simulink library "DQN_Lib (conflicted copy 2023-11-25 154811)"  (R2023b)
settings: Solver=VariableStepAuto  StartTime=0.0  StopTime=10.0  RelTol=1e-3
undefined symbols (not defined in the file): FreqRad, HrmOrd, Init, La, N, R, Ra, TimeStep, Ts, Ts_dqn, Ws
libraries: $bdroot x4, spsMeanVariableFrequencyLib x4, eeTransforms x3, spsabctodq0Lib x2, spsAlphaBetaZerotodq0Lib x1
(part 1 of 8)
settings Model: Creator=Robert  LastModifiedBy=rober
settings DebuggingCC: UnconnectedInputMsg=warning  UnconnectedOutputMsg=warning  UnconnectedLineMsg=warning
settings ModelReferenceCC: EnableRefExpFcnMdlSchedulingChecks=on
settings RTWCC: DLArmComputeVersion=19.05

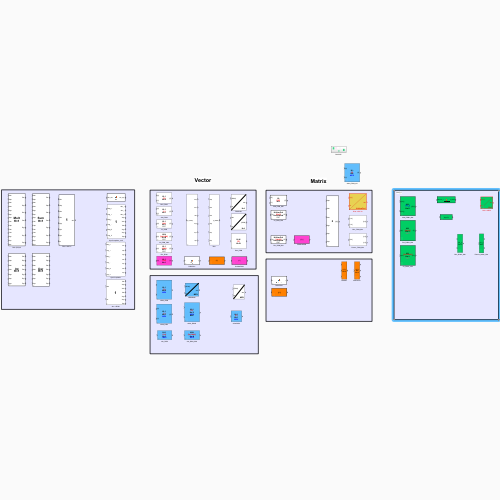
[thumbnail: Simulink's stored preview of the top-level diagram]
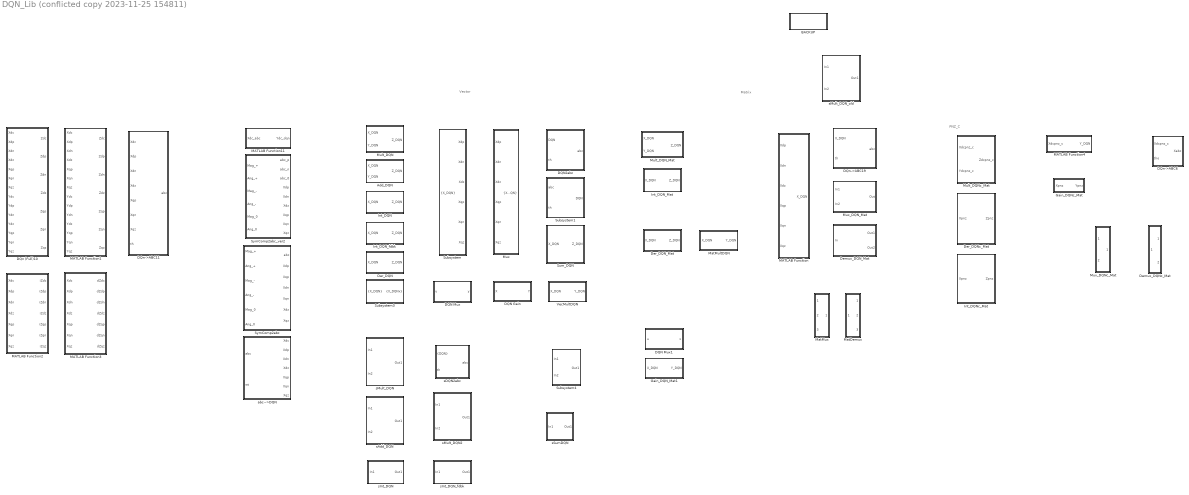
== system DQN_Lib (conflicted copy 2023-11-25 154811) ==
  note: PNZ_C
  note: Vector
  note: Matrix
  Add_DQN : Subsystem  mask{HrmOrd=1, chkHrmLst=off, HrmLst=[1]}
      mask prompts: HrmOrd "Harmonic order:"; chkHrmLst "Only specific harmonics"; HrmLst "Harmonic list:"
      mask Callback chkHrmLst:
      | EMT = get_param(gcb,'chkHrmLst');
      | 
      | if(strcmp(EMT,'on'))
      |    set_param(gcb,'MaskVisibilities',{'on','on','on'});
      | else
      |    set_param(gcb,'MaskVisibilities',{'on','on','off'});
      | end
      mask Display:
      | %plot([0 1])
      | port_label('input',1,'{X}');
      | port_label('input',2,'{Y}');
      | port_label('output',1,'{Z}');
      | 
      | 
      | 
      | harm = get_param(gcb, 'HrmOrd');
      | disp(['{\color{black}\bf\fontsize{12}Hi:',(harm),'}',newline,'{\color{red}\bf\fontsize{12}\{+\}}',newline,'{\color{black}\bf\fontsize{12}Ho:',(harm),'}'], 'texmode','on');
  BACKUP : Subsystem
  DQN Gain : MATLAB Function  TreatAsAtomicUnit=on  mask{H=1, Rvec=[]}
      mask prompts: H "Harmonic order:"; Rvec "[Ca,Cb,Cc]"
  DQN Mux : MATLAB Function  TreatAsAtomicUnit=on  mask{N=1}
      mask prompts: N "Harmonic order:"
  DQN Mux1 : MATLAB Function  TreatAsAtomicUnit=on  mask{N=1}
      mask prompts: N "Harmonic order:"
  DQN2abc : Subsystem  mask{HrmOrd=1}
      mask prompts: HrmOrd "Harmonic order:"
      mask Display:
      | plot([0 1], [0,1])
      | port_label('input',1,'{DQN}');
      | port_label('input',2,'wt');
      | port_label('output',1,'abc');
      | 
      | 
      | 
      | harm = get_param(gcb, 'HrmOrd');
      | %disp([newline,'{\bf\fontsize{12}H=',harm,'}'], 'texmode','on');
      | text(.95,.05,[newline,'{\bf\fontsize{12}H=',harm,'}'], 'horizontalAlignment', 'right', 'verticalAlignment','bottom','texmode','on')
  DQn (Full)10 : MATLAB Function  TreatAsAtomicUnit=on  mask{N=1}
      mask prompts: N "Harmonic order:"
  DQn->ABC11 : MATLAB Function  TreatAsAtomicUnit=on  mask{N=1}
      mask prompts: N "Harmonic order:"
  DQn->ABC19 : MATLAB Function  TreatAsAtomicUnit=on  mask{N=HrmOrd}
      mask prompts: N "Harmonic order:"
  DQn->ABC6 : MATLAB Function  TreatAsAtomicUnit=on  mask{N=1}
      mask prompts: N "Harmonic order:"
  Demux_DQN_Mat : Subsystem  mask{nrOut=2, N=0}
      mask prompts: nrOut "Number of outputs:"; N "Harmonic order:"
      mask init:
      | %fieldnames(get_param('DQn_ABC_Test_compact/Mux34','DialogParameters'))
      | 
      | if(nrOut==0)
      |     Simulink.SubSystem.deleteContents(gcb);
      | else
      | 
      |     PortHandles = get_param(gcb,'PortHandles');
      |     lenInp = length(PortHandles.Outport);
      |     
      |     if(nrOut ~= lenInp)
      | 
      | %         ss_size = ['[6,',num2str(nrOut),'*(',num2str(N+1),')]' ];
      | %         in_size = ['[',num2str(N+1),',6]'];
      | %         out_size = ['[',num2str(nrOut*(N+1)),',6]'];
      |         
      |         out_size = ['[',num2str(N+1),',6]' ];
      |         in_size = ['[',num2str(nrOut*(N+1)),',6]'];
      |         ss_size = ['[6,',num2str(N+1),']' ];
      |         
      |               
      |         Simulink.SubSystem.deleteContents(gcb);
      |         
      |         InportName = 'In';
      |         add_block('built-in/Inport',[gcb,'/',InportName] );
      |         set_param([gcb,'/', InportName ],'position' , [50,65+1*50,90,85+1*50]);
      |                
      |         add_block('simulink/Signal Attributes/Signal Specification', [gcb,'/','Sp_out'], 'Dimensions', in_size );
      |         set_param([gcb,'/','Sp_out'],'position' , [50,65+1*50,90,85+1*50]+[100,0,100,0]);
      |         
      |         add_block('simulink/Quick Insert/Math Operations/Transpose', [gcb,'/Transpose']);
      |         set_param([gcb,'/Transpose'],'position' , [50,65+1*50,90,85+1*50]+[200,0,200,0]);
      |         
      |         add_block('simulink/Math Operations/Reshape', [gcb,'/ss_block'])
      |         set_param([gcb,'/ss_block'],'position' , [50,65+1*50,90,85+1*50]+[300,0,300,0]);
      |        
      |         add_block('built-in/Demux',[gcb,'/Demux'], 'Outputs',num2str(nrOut));
      |         set_param([gcb,'/Demux'],'position' , [200,100,210,100+nrOut*50]+1*[300,0,300,0])
      |         
      |         add_line(gcb,'In/1', 'Sp_out/1','autorouting','on');
      |         add_line(gcb,'Sp_out/1', 'Transpose/1','autorouting','on');
      |         add_line(gcb,'Transpose/1', 'ss_block/1','autorouting','on');
      |         add_line(gcb,'ss_block/1', 'Demux/1','autorouting','on');
      |         
      |         MuxInputs = ['['];
      | 
      |         for i = 1 : nrOut
      |             MuxInputs = [MuxInputs,num2str((N+1)*6),','];
      |             OutportName = strcat('Out',num2str(i));
      |             ReshapeName = strcat('Re_out',num2str(i));
      |             TransposeName = strcat('Tr_out',num2str(i));
      |             SignalSpecName = strcat('Sp_out',num2str(i));
      | 
      |             add_block('built-in/Outport',[gcb,'/',OutportName] );
      |             set_param([gcb,'/', OutportName ],'position' , [750,65+i*50,790,85+i*50]+4*[100,0,100,0]);
      |                        
      |             add_block('simulink/Math Operations/Reshape',[gcb,'/',ReshapeName ], 'OutputDimensionality', 'Customize', 'OutputDimensions',ss_size );
      |             set_param([gcb,'/',ReshapeName ],'position' , [750,65+i*50,790,85+i*50]+1*[100,0,100,0]);
      |             
      |             add_block('simulink/Quick Insert/Math Operations/Transpose', [gcb,'/',TransposeName] );
      |             set_param([gcb,'/',TransposeName],'position' , [750,65+i*50,790,85+i*50]+2*[100,0,100,0]);
      |             
      |             add_block('simulink/Signal Attributes/Signal Specification', [gcb,'/',SignalSpecName], 'Dimensions', out_size );
      |             set_param([gcb,'/',SignalSpecName],'position', [750,65+i*50,790,85+i*50]+3*[100,0,100,0]);
      | 
      |             add_line(gcb,strcat('Demux/',num2str(i)), strcat(ReshapeName,'/1'), 'autorouting','on');
      |             add_line(gcb,strcat(ReshapeName,'/1'), strcat(TransposeName,'/1'),'autorouting','on');
      |             add_line(gcb,strcat(TransposeName,'/1'),strcat(SignalSpecName,'/1'),'autorouting','on');
      |             add_line(gcb,strcat(SignalSpecName,'/1'),strcat(OutportName,'/1'),'autorouting','on');
      |         end
      | 
      |         MuxInputs = [MuxInputs(1:end-1),']'];
      |         set_param([gcb,'/Demux'],'Outputs', MuxInputs);
      |         
      | 
      | 
      |     end
      | end
      mask Display:
      | NN = get_param(gcb, 'N');
      | 
      | 
      | Test = str2num(get_param(gcb, 'N'));
      | 
      | if(isempty(Test))
      |     std = ['[(N+1),6]'];
      |     text = [];
      |     for i = 1 : nrOut
      |         port_label('output',i,std);
      |     end
      |     port_label('input',1,['[',num2str(nrOut),'*(N+1),6]']);
      | else
      |     harm = str2num(NN);
      |     std = ['[',num2str(harm+1),',6]'];
      |     text = [];
      |     for i = 1 : nrOut
      |         port_label('output',i,std);
      |     end
      |     port_label('input',1,['[',num2str(nrOut*(harm+1)),',6]']);
      | end
  Demux_DQNc_Mat : Subsystem  mask{nrOut=2}
      mask prompts: nrOut "Number of outputs [{C}]"
      mask init:
      | if(isempty(nrOut))
      |     Simulink.SubSystem.deleteContents(gcb);
      | else
      | 
      |     IndexOptionArray = cell(2,1);
      |     IndexOptionArray(1) = {'Select all'           };
      |     IndexOptionArray(2) = {'Index vector (dialog)'};
      | 
      |     PortHandles = get_param(gcb,'PortHandles');
      | 
      |     lenOut = length(PortHandles.Outport);
      | 
      |     if(nrOut ~= lenOut) % Important to avoid reinitialization of the block!
      | 
      |         Simulink.SubSystem.deleteContents(gcb);
      | 
      |         add_block('built-in/Inport',[gcb,strcat('/In',num2str(1))]);
      |         set_param([gcb,strcat('/In',num2str(1))],'position' , [50,65+1*50,90,85+1*50]);
      | 
      |         for i = 1 : nrOut
      |             add_block('simulink/Signal Routing/Selector',[gcb,strcat('/Sel',num2str(i))],...
      |                 'IndexOptionArray',IndexOptionArray,...
      |                 'NumberOfDimensions','2',...
      |                 'IndexOptions','Index vector (dialog),Select all',...
      |                 'Indices',strcat(num2str((i-1)*3+1),':',num2str((i-1)*3+3),', 1') ...
      |                 );
      |             set_param([gcb,strcat('/Sel',num2str(i))],'position' , [450,65+i*50,490,85+i*50])
      | 
      | 
      |             add_block('built-in/Outport',[gcb,strcat('/Out',num2str(i))]);
      |             set_param([gcb,strcat('/Out',num2str(i))],'position' , [750,65+i*50,790,85+i*50]);
      | 
      |             add_line(gcb,strcat('In',num2str(1),'/1'),  strcat('Sel',num2str(i),'/1'),'autorouting','on');
      |             add_line(gcb,strcat('Sel',num2str(i),'/1'), strcat('Out',num2str(i),'/1'),'autorouting','on');
      |         end
      | 
      |     end
      | 
      | end
      mask Display: disp(['{\color{red}\bf\fontsize{12}} [\{X_C\}]',newline,' MUX'], 'texmode','on');
  Der_DQN : Subsystem  mask{HrmOrd=1, FreqRad=2*pi*50, Ts=0, EMT=on, sw_soft=on, chkHrmLst=off, HrmLst=[1]}
      mask prompts: HrmOrd "Harmonic order:"; FreqRad "Angular frequency (rad/s);"; Ts "Time step (s):"; EMT "Enable EMT"; sw_soft "Soft start"; chkHrmLst "Only specific harmonics"; HrmLst "Harmonic list:"
      mask Callback EMT:
      | EMT = get_param(gcb,'EMT');
      | EMT2 = get_param(gcb,'chkHrmLst');
      | 
      | 
      | if(strcmp(EMT,'on') && strcmp(EMT2,'on'))
      |    set_param(gcb,'MaskVisibilities',{'on','on','on','on','on','on','on'});
      | elseif(strcmp(EMT,'on') && strcmp(EMT2,'off'))
      |    set_param(gcb,'MaskVisibilities',{'on','on','on','on','on','on','off'});
      | elseif(strcmp(EMT,'off') && strcmp(EMT2,'on'))
      |    set_param(gcb,'MaskVisibilities',{'on','on','on','on','off','on','on'});
      | else
      |    set_param(gcb,'MaskVisibilities',{'on','on','on','on','off','on','off'});
      | end
      mask Callback chkHrmLst:
      | EMT = get_param(gcb,'EMT');
      | EMT2 = get_param(gcb,'chkHrmLst');
      | 
      | 
      | if(strcmp(EMT,'on') && strcmp(EMT2,'on'))
      |    set_param(gcb,'MaskVisibilities',{'on','on','on','on','on','on','on'});
      | elseif(strcmp(EMT,'on') && strcmp(EMT2,'off'))
      |    set_param(gcb,'MaskVisibilities',{'on','on','on','on','on','on','off'});
      | elseif(strcmp(EMT,'off') && strcmp(EMT2,'on'))
      |    set_param(gcb,'MaskVisibilities',{'on','on','on','on','off','on','on'});
      | else
      |    set_param(gcb,'MaskVisibilities',{'on','on','on','on','off','on','off'});
      | end
      mask Display:
      | %plot([0 1])
      | port_label('input',1,'{X}');
      | port_label('output',1,'{Z}');
      | 
      | harm = get_param(gcb, 'HrmOrd');
      | 
      | if(numel(get_param(gcb, 'EMT'))==2)
      |     disp(['{\color{black}\bf\fontsize{12}Hi:',(harm),'}',newline,'{\color{red}\bf\fontsize{12}\{d/dt\}}',newline,'{\color{black}\bf\fontsize{12}Ho:',(harm),'}',newline,'{\color{gray}\bf\fontsize{12}EMT}'], 'texmode','on');
      | else
      |     disp(['{\color{black}\bf\fontsize{12}Hi:',(harm),'}',newline,'{\color{red}\bf\fontsize{12}\{d/dt\}}',newline,'{\color{black}\bf\fontsize{12}Ho:',(harm),'}'], 'texmode','on');
      | end
  Der_DQN_Mat : MATLAB Function  TreatAsAtomicUnit=on  mask{N=HrmOrd, w=FreqRad, Ts=Ts, EMT=on, sw_soft=on}
      mask prompts: N "Harmonic order:"; w "Frequency (rad/s):"; Ts "Time step (s):"; EMT "Enable EMT"; sw_soft "Soft start?"
  Der_DQNc_Mat : MATLAB Function  TreatAsAtomicUnit=on  mask{Ts=50e-6, N=1, w=2*pi*50, EMT=on, sw_soft=on}
      mask prompts: Ts "Time step (s):"; N "Harmonic order:"; w "Angular frequency [1/rad]:"; sw_soft "Soft start"
  Gain_DQN_Mat1 : MATLAB Function  TreatAsAtomicUnit=on  mask{H=1, R=[], chkInv=off}
      mask prompts: H "Harmonic order:"; R "Line matrix [3x3]"; chkInv "Invert?"
  Gain_DQNc_Mat : MATLAB Function  TreatAsAtomicUnit=on  mask{Rabc=[R zeros(3,3); zeros(3,3) R], HRM=N, chkInv=off}
      mask prompts: Rabc "Line matrix [3x3]:"; HRM "Harmonic order:"; chkInv "Invert"
  Int_DQN : Subsystem  mask{HrmOrd=1, FreqRad=2*pi*50, TimeStep=50e-6, Init=zeros(1,6), EMT=on, chkHrmLst=off, HrmLst=[1]}
      mask prompts: HrmOrd "Harmonic order:"; FreqRad "Angular frequency (rad/s);"; TimeStep "Time step (s):"; Init "DC init [1x6]:"; EMT "Enable EMT"; chkHrmLst "Only specific harmonics"; HrmLst "Harmonic list:"
      mask Callback chkHrmLst:
      | EMT = get_param(gcb,'chkHrmLst');
      | 
      | if(strcmp(EMT,'on'))
      |    set_param(gcb,'MaskVisibilities',{'on','on','on','on','on','on','on'});
      | else
      |    set_param(gcb,'MaskVisibilities',{'on','on','on','on','on','on','off'});
      | end
      mask Display:
      | %plot([0 1])
      | port_label('input',1,'{X}');
      | port_label('output',1,'{Z}');
      | 
      | harm = get_param(gcb, 'HrmOrd');
      | 
      | if(numel(get_param(gcb, 'EMT'))==2)
      |     disp(['{\color{black}\bf\fontsize{12}Hi:',(harm),'}',newline,'{\color{red}\bf\fontsize{12}\{Int\}}',newline,'{\color{black}\bf\fontsize{12}Ho:',(harm),'}',newline,'{\color{gray}\bf\fontsize{12}EMT}'], 'texmode','on');
      | else
      |     disp(['{\color{black}\bf\fontsize{12}Hi:',(harm),'}',newline,'{\color{red}\bf\fontsize{12}\{Int\}}',newline,'{\color{black}\bf\fontsize{12}Ho:',(harm),'}'], 'texmode','on');
      | end
  Int_DQN_Mat : MATLAB Function  TreatAsAtomicUnit=on  mask{N=HrmOrd, dt=TimeStep, w=FreqRad, EMT=on, InitInt=Init}
      mask prompts: N "Order number:"; dt "Time step (s):"; w "Angular frequency (1/rad):"; InitInt "Initial conditions [1x6]:"
  Int_DQN_fdbk : Subsystem  mask{HrmOrd=N, FreqRad=Ws, TimeStep=Ts_dqn, swFeed=on, R=Ra, iL=1/La}
      mask prompts: HrmOrd "Harmonic order:"; FreqRad "Angular frequency (rad/s);"; TimeStep "Time step (s):"; swFeed "Enable feedback"; R "Feedback parameter (Kr):"; iL "Integrator parameter (Kl):"
      mask Callback swFeed:
      | EMT = get_param(gcb,'swFeed');
      | 
      | if(strcmp(EMT,'on'))
      |    set_param(gcb,'MaskVisibilities',{'on','on','on','on','on','on'});
      | else
      |    set_param(gcb,'MaskVisibilities',{'on','on','on','on','off','off'});
      | end
      mask Display:
      | %plot([0 1])
      | port_label('input',1,'{X}');
      | port_label('output',1,'{Z}');
      | 
      | harm = get_param(gcb, 'HrmOrd');
      | disp(['{\color{black}\bf\fontsize{12}Hi:',(harm),'}',newline,'{\color{red}\bf\fontsize{12}\{Int-fdbk\}}',newline,'{\color{black}\bf\fontsize{12}Ho:',(harm),'}',newline,'{\color{gray}\bf\fontsize{12}EMT}'], 'texmode','on');
  Int_DQNc_Mat : MATLAB Function  TreatAsAtomicUnit=on  mask{N=1, dt=50e-6, w=2*pi*50, InitInt=zeros(3,1), swFeed=on, R=eye(3), iL=eye(3)}
      mask prompts: N "Order number:"; dt "Time step (s):"; w "Angular frequency (1/rad):"; InitInt "Initial conditions DC [3x1]:"; swFeed "Enable feedback"; R "Feedback parameter (Kr {abc}):"; iL "Feedback parameter (Ki {abc}):"
  MATLAB Function : MATLAB Function  TreatAsAtomicUnit=on  mask{N=0}
      mask prompts: N "Harmonic order:"
  MATLAB Function1 : MATLAB Function  TreatAsAtomicUnit=on  mask{N=1}
      mask prompts: N "Harmonic order:"
  MATLAB Function11 : MATLAB Function  TreatAsAtomicUnit=on
  MATLAB Function2 : MATLAB Function  TreatAsAtomicUnit=on  mask{N=1, w=2*pi*50, Ts=50e-6, IntDC=on}
      mask prompts: N "Harmonic order:"; w "Frequency (rad/s):"; Ts "Time step (s):"; IntDC "Integrate Xdc?"
  MATLAB Function3 : MATLAB Function  TreatAsAtomicUnit=on  mask{N=1, w=2*pi*50, Ts=0, EMT=0}
      mask prompts: N "Harmonic order:"; w "Frequency (rad/s):"; Ts "Time step (s):"; EMT "Enable EMT"
  MATLAB Function4 : MATLAB Function  TreatAsAtomicUnit=on
  MatDemux : Subsystem  mask{nrOut=3}
      mask prompts: nrOut "Number of outputs [{C}]"
      mask init:
      | if(isempty(nrOut))
      |     Simulink.SubSystem.deleteContents(gcb);
      | else
      | 
      |     IndexOptionArray = cell(2,1);
      |     IndexOptionArray(1) = {'Select all'           };
      |     IndexOptionArray(2) = {'Index vector (dialog)'};
      | 
      |     PortHandles = get_param(gcb,'PortHandles');
      | 
      |     lenOut = length(PortHandles.Outport);
      | 
      |     if(nrOut ~= lenOut) % Important to avoid reinitialization of the block!
      | 
      |         Simulink.SubSystem.deleteContents(gcb);
      | 
      |         add_block('built-in/Inport',[gcb,strcat('/In',num2str(1))]);
      |         set_param([gcb,strcat('/In',num2str(1))],'position' , [50,65+1*50,90,85+1*50]);
      | 
      |         for i = 1 : nrOut
      |             add_block('simulink/Signal Routing/Selector',[gcb,strcat('/Sel',num2str(i))],...
      |                 'IndexOptionArray',IndexOptionArray,...
      |                 'NumberOfDimensions','2',...
      |                 'IndexOptions','Select all,Index vector (dialog)',...
      |                 'Indices',strcat('1,',num2str((i-1)*6+1),':',num2str((i-1)*6+6)) );
      |             set_param([gcb,strcat('/Sel',num2str(i))],'position' , [450,65+i*50,490,85+i*50])
      | 
      | 
      |             add_block('built-in/Outport',[gcb,strcat('/Out',num2str(i))]);
      |             set_param([gcb,strcat('/Out',num2str(i))],'position' , [750,65+i*50,790,85+i*50]);
      | 
      |             add_line(gcb,strcat('In',num2str(1),'/1'),  strcat('Sel',num2str(i),'/1'),'autorouting','on');
      |             add_line(gcb,strcat('Sel',num2str(i),'/1'), strcat('Out',num2str(i),'/1'),'autorouting','on');
      |         end
      | 
      |     end
      | 
      | end
      mask Display: disp(['{\color{red}\bf\fontsize{12}} [\{C\}]',newline,'  DE-',newline,' MUX'], 'texmode','on');
  MatMultDQN : MATLAB Function  TreatAsAtomicUnit=on  mask{H=1, R=[], chkInv=off}
      mask prompts: H "Harmonic order:"; R "Line matrix [3x3]"; chkInv "Invert?"
  MatMux : Subsystem  mask{nrInp=3}
      mask prompts: nrInp "Number of inputs [{C}]"
      mask init:
      | %blocks = find_system(gcb,'LookUnderMasks','on','FollowLinks','on')
      | %set_param(gcb, 'MaskSelfModifiable', 'on');
      | 
      | % if(SSM == [])
      | %     Simulink.SubSystem.deleteContents(gcb);
      | % else
      | 
      | if(isempty(nrInp))
      |     Simulink.SubSystem.deleteContents(gcb);
      | else
      | 
      |     nrOut = 1;
      | 
      | 
      | PortHandles = get_param(gcb,'PortHandles');
      | lenInp = length(PortHandles.Inport);
      | lenOut = length(PortHandles.Inport);
      | 
      | if(nrInp ~= lenInp)
      |     %disp('ENTERED')
      |     Simulink.SubSystem.deleteContents(gcb);
      | %     add_block('simulink/Continuous/State-Space', [gcb,'/ss_block'], 'A','SS.A', 'B','SS.B', 'C','SS.C', 'D','SS.D', 'X0','X0')
      | %     set_param([gcb,'/ss_block'],'position' , [350,100,450,150])
      | 
      | 
      | 
      |         add_block('simulink/Math Operations/Matrix Concatenate',[gcb,'/Mux'], 'NumInputs',num2str(nrInp), 'ConcatenateDimension',num2str(2));
      |         set_param([gcb,'/Mux'],'position' , [200,100,250,100+nrInp*50])
      |         
      | %         add_block('built-in/Demux',[gcb,'/Demux'], 'Outputs',num2str(nrOut));
      | %         set_param([gcb,'/Demux'],'position' , [500,100,550,100+nrOut*50])
      | 
      | 
      |         for i = 1 : nrInp
      |             add_block('built-in/Inport',[gcb,strcat('/In',num2str(i))]);
      |             set_param([gcb,strcat('/In',num2str(i))],'position' , [50,65+i*50,90,85+i*50]);
      |             add_line(gcb,strcat('In',num2str(i),'/1'),strcat('Mux/',num2str(i)),'autorouting','on');
      |         end
      | 
      |         for i = 1 : nrOut
      |             add_block('built-in/Outport',[gcb,strcat('/Out',num2str(i))]);
      |             set_param([gcb,strcat('/Out',num2str(i))],'position' , [750,65+i*50,790,85+i*50]);
      |             add_line(gcb,strcat('Mux/',num2str(i)), strcat('Out',num2str(i),'/1'),'autorouting','on');
      |         end
      | 
      | 
      | %     add_line(gcb, 'Mux/1', 'ss_block/1')
      | %     add_line(gcb, 'ss_block/1', 'Demux/1')
      | 
      | end
      | 
      | end
      mask Display: disp(['{\color{red}\bf\fontsize{12}} [\{C\}]',newline,' MUX'], 'texmode','on');
  Mult_DQN : Subsystem  mask{HrmOrd=1, HrmDbl=on, chkHrmLst=off, HrmLstX=[1], HrmLstY=[1]}
      mask prompts: HrmOrd "Harmonic order:"; HrmDbl "Double harmonic"; chkHrmLst "Only specific harmonics"; HrmLstX "Harmonic list X:"; HrmLstY "Harmonic list Y:"
      mask Callback chkHrmLst:
      | EMT = get_param(gcb,'chkHrmLst');
      | 
      | if(strcmp(EMT,'on'))
      |    set_param(gcb,'MaskVisibilities',{'on','on','on','on','on'});
      | else
      |    set_param(gcb,'MaskVisibilities',{'on','on','on','off','off'});
      | end
      mask Display:
      | %plot([0 1])
      | port_label('input',1,'{X}');
      | port_label('input',2,'{Y}');
      | port_label('output',1,'{Z}');
      | 
      | 
      | 
      | harm = str2num(get_param(gcb, 'HrmOrd'));
      | HrmDbl = get_param(gcb, 'HrmDbl');
      | if(HrmDbl=="on")
      |     disp(['{\color{black}\bf\fontsize{12}Hi:',num2str(harm),'}',newline,'{\color{red}\bf\fontsize{12}\{X\}}',newline,'{\color{black}\bf\fontsize{12}Ho:',num2str(2*harm),'}'], 'texmode','on');
      | else
      |     disp(['{\color{black}\bf\fontsize{12}Hi:',num2str(harm),'}',newline,'{\color{red}\bf\fontsize{12}\{X\}}',newline,'{\color{black}\bf\fontsize{12}Ho:',num2str(harm),'}'], 'texmode','on');
      | end
      | 
      | 
      | %text(.95,.05,[newline,'{\bf\fontsize{12}H=',harm,'}'], 'horizontalAlignment', 'right', 'verticalAlignment','bottom','texmode','on')
  Mult_DQN_Mat : MATLAB Function  TreatAsAtomicUnit=on  mask{N=HrmOrd, HrmDbl=on}
      mask prompts: N "Harmonic order:"; HrmDbl "Double Harmonic"
  Mult_DQNc_Mat : MATLAB Function  TreatAsAtomicUnit=on  mask{N=1, HrmDbl=on}
      mask prompts: N "Harmonic order:"; HrmDbl "Double Harmonic"
  Mux : Subsystem  mask{N=1}
      mask prompts: N "Harmonic order:"
  Mux_DQN_Mat : Subsystem  mask{nrInp=2, N=0}
      mask prompts: nrInp "Number of inputs:"; N "Harmonic order:"
      mask init:
      | %fieldnames(get_param('DQn_ABC_Test_compact/Mux34','DialogParameters'))
      | 
      | if(nrInp==0)
      |     Simulink.SubSystem.deleteContents(gcb);
      | else
      | 
      |     PortHandles = get_param(gcb,'PortHandles');
      |     lenInp = length(PortHandles.Inport);
      |     lenOut = length(PortHandles.Inport);
      |     
      |     if(nrInp ~= lenInp)
      | 
      |         ss_size = ['[6,',num2str(nrInp),'*(',num2str(N+1),')]' ];
      |         in_size = ['[',num2str(N+1),',6]'];
      |         out_size = ['[',num2str(nrInp*(N+1)),',6]'];
      |         
      |         Simulink.SubSystem.deleteContents(gcb);
      |         add_block('simulink/Math Operations/Reshape', [gcb,'/ss_block'], 'OutputDimensionality', 'Customize', 'OutputDimensions', ss_size)
      |         set_param([gcb,'/ss_block'],'position' , [350,100,450,150]+[300,0,300,0])
      | 
      | 
      |         add_block('built-in/Mux',[gcb,'/Mux'], 'Inputs',num2str(nrInp));
      |         set_param([gcb,'/Mux'],'position' , [200,100,250,100+nrInp*50]+[300,0,300,0])
      |         
      |         MuxInputs = ['['];
      | 
      |         for i = 1 : nrInp
      |             MuxInputs = [MuxInputs,num2str((N+1)*6),','];
      |             InportName = strcat('In',num2str(i));
      |             ReshapeName = strcat('Re_in',num2str(i));
      |             TransposeName = strcat('Tr_in',num2str(i));
      |             SignalSpecName = strcat('Sp_in',num2str(i));
      | 
      |             add_block('built-in/Inport',[gcb,'/',InportName] );
      |             set_param([gcb,'/', InportName ],'position' , [50,65+i*50,90,85+i*50]);
      |             
      |             add_block('simulink/Signal Attributes/Signal Specification', [gcb,'/',SignalSpecName], 'Dimensions', in_size );
      |             set_param([gcb,'/',SignalSpecName],'position' , [50,65+i*50,90,85+i*50]+[100,0,100,0]);
      |             
      |             add_block('simulink/Quick Insert/Math Operations/Transpose', [gcb,'/',TransposeName] );
      |             set_param([gcb,'/',TransposeName],'position' , [50,65+i*50,90,85+i*50]+[200,0,200,0]);
      |             
      |             add_block('simulink/Math Operations/Reshape',[gcb,'/',ReshapeName ]);
      |             set_param([gcb,'/',ReshapeName ],'position' , [50,65+i*50,90,85+i*50]+[300,0,300,0]);
      | 
      |             add_line(gcb,strcat(InportName,'/1'), strcat(SignalSpecName,'/1'), 'autorouting','on');
      |             add_line(gcb,strcat(SignalSpecName,'/1'), strcat(TransposeName,'/1'), 'autorouting','on');
      |             add_line(gcb,strcat(TransposeName,'/1'), strcat(ReshapeName,'/1'), 'autorouting','on');
      |             add_line(gcb,strcat(ReshapeName,'/1'),strcat('Mux/',num2str(i)),'autorouting','on');
      | 
      |         end
      |         MuxInputs = [MuxInputs(1:end-1),']'];
      |         set_param([gcb,'/Mux'],'Inputs', MuxInputs);
      |         
      |         add_block('simulink/Signal Attributes/Signal Specification', [gcb,'/','Sp_out'], 'Dimensions', out_size );
      |         set_param([gcb,'/','Sp_out'],'position' , [750,65+1*50,790,85+1*50]+[200,0,200,0]);
      | 
      |         add_block('built-in/Outport',[gcb,'/Out']);
      |         set_param([gcb,'/Out'],'position' , [750,65+1*50,790,85+1*50]+[300,0,300,0]);
      |         add_line(gcb,'Mux/1','ss_block/1','autorouting','on');
      | 
      |         add_block('simulink/Quick Insert/Math Operations/Transpose', [gcb,'/Transpose']);
      |         set_param([gcb,'/Transpose'],'position' , [750,65+1*50,790,85+1*50]+[100,0,100,0]);
      |         
      |         
      |         add_line(gcb,'ss_block/1', 'Transpose/1','autorouting','on');
      |         add_line(gcb,'Transpose/1', 'Sp_out/1','autorouting','on');
      |         add_line(gcb,'Sp_out/1', 'Out/1','autorouting','on');
      | 
      |     end
      | end
      mask Display:
      | NN = get_param(gcb, 'N');
      | 
      | 
      | Test = str2num(get_param(gcb, 'N'));
      | 
      | if(isempty(Test))
      |     std = ['[(N+1),6]'];
      |     text = [];
      |     for i = 1 : nrInp
      |         port_label('input',i,std);
      |     end
      |     port_label('output',1,['[',num2str(nrInp),'*(N+1),6]']);
      | else
      |     harm = str2num(NN);
      |     std = ['[',num2str(harm+1),',6]'];
      |     text = [];
      |     for i = 1 : nrInp
      |         port_label('input',i,std);
      |     end
      |     port_label('output',1,['[',num2str(nrInp*(harm+1)),',6]']);
      | end
  Mux_DQNc_Mat : Subsystem  mask{nrInp=2}
      mask prompts: nrInp "Number of inputs [{C}]"
      mask init:
      | %blocks = find_system(gcb,'LookUnderMasks','on','FollowLinks','on')
      | %set_param(gcb, 'MaskSelfModifiable', 'on');
      | 
      | % if(SSM == [])
      | %     Simulink.SubSystem.deleteContents(gcb);
      | % else
      | 
      | if(isempty(nrInp))
      |     Simulink.SubSystem.deleteContents(gcb);
      | else
      | 
      |     nrOut = 1;
      | 
      | 
      | PortHandles = get_param(gcb,'PortHandles');
      | lenInp = length(PortHandles.Inport);
      | lenOut = length(PortHandles.Inport);
      | 
      | if(nrInp ~= lenInp)
      |     %disp('ENTERED')
      |     Simulink.SubSystem.deleteContents(gcb);
      | %     add_block('simulink/Continuous/State-Space', [gcb,'/ss_block'], 'A','SS.A', 'B','SS.B', 'C','SS.C', 'D','SS.D', 'X0','X0')
      | %     set_param([gcb,'/ss_block'],'position' , [350,100,450,150])
      | 
      | 
      | 
      |         add_block('simulink/Math Operations/Matrix Concatenate',[gcb,'/Mux'], 'NumInputs',num2str(nrInp), 'ConcatenateDimension',num2str(1));
      |         set_param([gcb,'/Mux'],'position' , [200,100,250,100+nrInp*50])
      |         
      | %         add_block('built-in/Demux',[gcb,'/Demux'], 'Outputs',num2str(nrOut));
      | %         set_param([gcb,'/Demux'],'position' , [500,100,550,100+nrOut*50])
      | 
      | 
      |         for i = 1 : nrInp
      |             add_block('built-in/Inport',[gcb,strcat('/In',num2str(i))]);
      |             set_param([gcb,strcat('/In',num2str(i))],'position' , [50,65+i*50,90,85+i*50]);
      |             add_line(gcb,strcat('In',num2str(i),'/1'),strcat('Mux/',num2str(i)),'autorouting','on');
      |         end
      | 
      |         for i = 1 : nrOut
      |             add_block('built-in/Outport',[gcb,strcat('/Out',num2str(i))]);
      |             set_param([gcb,strcat('/Out',num2str(i))],'position' , [750,65+i*50,790,85+i*50]);
      |             add_line(gcb,strcat('Mux/',num2str(i)), strcat('Out',num2str(i),'/1'),'autorouting','on');
      |         end
      | 
      | 
      | %     add_line(gcb, 'Mux/1', 'ss_block/1')
      | %     add_line(gcb, 'ss_block/1', 'Demux/1')
      | 
      | end
      | 
      | end
      mask Display: disp(['{\color{red}\bf\fontsize{12}} [\{X_C\}]',newline,' MUX'], 'texmode','on');
  Subsystem : Subsystem  mask{N=1}
      mask prompts: N "Harmonic order:"
  Subsystem1 : Subsystem  mask{HrmOrd=1, Freq=0, Ts=50e-6}
      mask prompts: HrmOrd "Harmonic order:"; Freq "Frequency (Hz):"; Ts "Sample time (s):"
      mask Display:
      | plot([0 1], [0,1])
      | port_label('input',1,'abc');
      | port_label('input',2,'wt');
      | port_label('output',1,'{DQN}');
      | 
      | 
      | 
      | harm = get_param(gcb, 'HrmOrd');
      | %disp([newline,'{\bf\fontsize{12}H=',harm,'}'], 'texmode','on');
      | text(.95,.05,[newline,'{\bf\fontsize{12}H=',harm,'}'], 'horizontalAlignment', 'right', 'verticalAlignment','bottom','texmode','on')
  Subsystem3 : Subsystem  mask{HOI=1, HOO=1}
      mask prompts: HOI "Input harmonic order:"; HOO "Output harmonic order:"
      mask Display:
      | %plot([0 1])
      | port_label('input',1,'{X}');
      | port_label('output',1,'{Y}');
      | 
      | 
      | 
      | HOI = get_param(gcb, 'HOI');
      | HOO = get_param(gcb, 'HOO');
      | disp(['{\color{black}\bf\fontsize{12}Hi:',(HOI),'}',newline,'{\color{red}\bf\fontsize{12}Trim}',newline,'{\color{black}\bf\fontsize{12}Ho:',(HOO),'}'], 'texmode','on');
  Subsystem4 : Subsystem
      mask Display:
      | plot([0 1], [0,1])
      | port_label('input',1,'{DQN}');
      | port_label('input',2,'wt');
      | port_label('output',1,'abc');
      | 
      | text(.95,.05,[newline,'{\bf\fontsize{12}MEX}'], 'horizontalAlignment', 'right', 'verticalAlignment','bottom','texmode','on')
  Sum_DQN : Subsystem  mask{HrmOrd=N}
      mask prompts: HrmOrd "Harmonic order:"
      mask Display:
      | %plot([0 1])
      | %port_label('input',1,'{X}');
      | %port_label('output',1,'{Z}');
      | 
      | port_label('input',1,'');
      | port_label('output',1,'');
      | 
      | harm = get_param(gcb, 'HrmOrd');
      | disp(['{\color{black}\bf\fontsize{12}Hi:',(harm),'}',newline,'{\color{red}\bf\fontsize{12}\{\Sigma\}}',newline,'{\color{black}\bf\fontsize{12}Ho:',(harm),'}'], 'texmode','on');
      | 
      | radius = 1
      | 
      | 
      | rsq = radius * radius;
      | R = round(radius);
      | c = R + 1;
      | t = 2*R + 1;
      | y = zeros(t);
      | 
      | % points on St George's cross
      | y(:, c) = 1;
      | y(c, :) = 1;
      | 
      | for rstart = 1:R
      |     rend = round(sqrt(rsq - rstart * rstart));
      |     if rend < rstart
      |         break
      |     end
      | 
      |     % points on St Andrew's cross
      |     y(c+rstart, c+rstart) = 1;
      |     y(c+rstart, c-rstart) = 1;
      |     y(c-rstart, c+rstart) = 1;
      |     y(c-rstart, c-rstart) = 1;
      | 
      |     % fill in octants
      |     y(c+rstart:c+rend, c+rstart) = 1;
      |     y(c+rstart:c+rend, c-rstart) = 1;
      |     y(c-rend:c-rstart, c+rstart) = 1;
      |     y(c-rend:c-rstart, c-rstart) = 1;
      |     y(c+rstart, c+rstart:c+rend) = 1;
      |     y(c-rstart, c+rstart:c+rend) = 1;
      |     y(c+rstart, c-rend:c-rstart) = 1;
      |     y(c-rstart, c-rend:c-rstart) = 1;
      | end
  SymComp2abc : Subsystem  mask{H=1, f=50}
      mask prompts: H "Harmonic order:"; f "Frequency (1/s):"
  SymComp2abc_ver2 : Subsystem  mask{H=1, f=50}
      mask prompts: H "Harmonic order:"; f "Frequency (1/s):"
      mask Display:
      | port_label('input',1,'Mag_+');
      | port_label('input',2,'Ang_+');
      | port_label('input',3,'Mag_-');
      | port_label('input',4,'Ang_-');
      | port_label('input',5,'Mag_0');
      | port_label('input',6,'Ang_0');
      | 
      | 
      | port_label('output',1,'abc_+');
      | port_label('output',2,'abc_-');
      | port_label('output',3,'abc_0');
      | port_label('output',4,'Xdp');
      | port_label('output',5,'Xdn');
      | port_label('output',6,'Xdz');
      | port_label('output',7,'Xqp');
      | port_label('output',8,'Xqn');
      | port_label('output',9,'Xqz');
      | 
      | 
      | 
      | harm = get_param(gcb, 'H');
      | disp(['{\bf\fontsize{24}',harm,'}'], 'texmode','on');
  VecMultDQN : MATLAB Function  TreatAsAtomicUnit=on  mask{H=1, R=[], chkInv=off}
      mask prompts: H "Harmonic order:"; R "Line matrix [3x3]"; chkInv "Invert?"
  abc-->DQN : Subsystem  mask{H=1, f=50, Ts=Ts}
      mask prompts: H "Harmonic order:"; f "Frequency (Hz):"; Ts "Sample time (s):"
      mask Display:
      | port_label('input',1,'abc');
      | port_label('input',2,'wt');
      | 
      | port_label('output',1,'Xdc');
      | port_label('output',2,'Xdp');
      | port_label('output',3,'Xdn');
      | port_label('output',4,'Xdz');
      | port_label('output',5,'Xqp');
      | port_label('output',6,'Xqn');
      | port_label('output',7,'Xqz');
      | 
      | 
      | 
      | harm = get_param(gcb, 'H');
      | disp(['{\bf\fontsize{24}',harm,'}'], 'texmode','on');
  sAdd_DQN : Subsystem  mask{HRM=1}
      mask prompts: HRM "Harmonic order:"
      mask Display:
      | %plot([0 1])
      | port_label('input',1,'{X}');
      | port_label('input',2,'{Y}');
      | port_label('output',1,'{Z}');
      | 
      | 
      | 
      | %harm = (get_param(gcb, 'HRM'));
      | %disp(['{\color{black}\bf\fontsize{12}Hi:',num2str(harm),'}',newline,'{\color{red}\bf\fontsize{12}\{+\}}',newline,'{\color{black}\bf\fontsize{12}Ho:',num2str(harm),newline,'{\color{blue}\bf\fontsize{12}MEX}','}'], 'texmode','on');
      | harm = get_param(gcb, 'HRM');
      | disp(['{\color{black}\bf\fontsize{12}Hi:',(harm),'}',newline,'{\color{red}\bf\fontsize{12}\{+\}}',newline,'{\color{black}\bf\fontsize{12}Ho:',(harm),newline,'{\color{blue}\bf\fontsize{12}MEX}','}'], 'texmode','on');
  sDQN2abc : Subsystem  mask{HRM=1}
      mask prompts: HRM "Harmonic order:"
      mask Display:
      | plot([0 1], [0,1])
      | port_label('input',1,'{DQN}');
      | port_label('input',2,'wt');
      | port_label('output',1,'abc');
      | 
      | text(.95,.05,[newline,'{\bf\fontsize{12}MEX}'], 'horizontalAlignment', 'right', 'verticalAlignment','bottom','texmode','on')
  sInt_DQN : Subsystem  mask{HRM=1, Ws=2*pi*50, Ts=50e-6, HrmSeq=off}
      mask prompts: HRM "Harmonic order:"; Ws "Angular frequency (1/rad):"; Ts "Time step (s):"; HrmSeq "Pos. odd / neg. even harmonics (1p, 2n, 3p...)"
      mask Display:
      | %plot([0 1])
      | %port_label('input',1,'{X}');
      | %port_label('output',1,'{Z}');
      | 
      | port_label('input',1,'');
      | port_label('output',1,'');
      | 
      | harm = get_param(gcb, 'HRM');
      | 
      | disp(['{\color{black}\bf\fontsize{12}Hi:',(harm),'}',newline,'{\color{red}\bf\fontsize{12}\{Int\}}',newline,'{\color{black}\bf\fontsize{12}Ho:',(harm),'}',newline,'{\color{blue}\bf\fontsize{12}MEX}'], 'texmode','on');
  sInt_DQN_fdbk : Subsystem  mask{HRM=N, Ws=Ws, Ts=Ts, HrmSeq=off, swFeed=off, R=1, iL=1}
      mask prompts: HRM "Harmonic order:"; Ws "Angular frequency (1/rad):"; Ts "Time step (s):"; HrmSeq "Pos. odd / neg. even harmonics (1p, 2n, 3p...)"; swFeed "Enable feedback"; R "Feedback parameter (Kr):"; iL "Integrator parameter (Ki):"
      mask Callback swFeed:
      | EMT = get_param(gcb,'swFeed');
      | 
      | if(strcmp(EMT,'on'))
      |    set_param(gcb,'MaskVisibilities',{'on','on','on','on','on','on','on'});
      | else
      |    set_param(gcb,'MaskVisibilities',{'on','on','on','on','on','off','off'});
      | end
      mask Display:
      | %plot([0 1])
      | %port_label('input',1,'{X}');
      | %port_label('output',1,'{Z}');
      | 
      | port_label('input',1,'');
      | port_label('output',1,'');
      | 
      | harm = get_param(gcb, 'HRM');
      | 
      | disp(['{\color{black}\bf\fontsize{12}Hi:',(harm),'}',newline,'{\color{red}\bf\fontsize{12}\{Int-fdbk\}}',newline,'{\color{black}\bf\fontsize{12}Ho:',(harm),'}',newline,'{\color{blue}\bf\fontsize{12}MEX}'], 'texmode','on');
  sMult_DQN : Subsystem  mask{HRM=1, HrmDbl=on, HrmSeq=off}
      mask prompts: HRM "Harmonic order:"; HrmDbl "Double harmonic"; HrmSeq "Pos. odd / neg. even harmonics (1p, 2n, 3p...)"
      mask init:
      | if(HrmDbl == 0 && HrmSeq == 0)
      |     HrmOpt = 0;
      | elseif(HrmDbl == 1 && HrmSeq == 0)
      |     HrmOpt = 1;
      | elseif(HrmDbl == 0 && HrmSeq == 1)
      |     HrmOpt = 2;
      | elseif(HrmDbl == 1 && HrmSeq == 1)
      |     HrmOpt = 3;
      | end
      mask Display:
      | %plot([0 1])
      | %port_label('input',1,'{X}');
      | %port_label('input',2,'{Y}');
      | %port_label('output',1,'{Z}');
      | 
      | port_label('input',1,'');
      | port_label('input',2,'');
      | port_label('output',1,'');
      | 
      | 
      | harm = str2num(get_param(gcb, 'HRM'));
      | HrmDbl = get_param(gcb, 'HrmDbl');
      | if(HrmDbl=="on")
      |     disp(['{\color{black}\bf\fontsize{12}Hi:',num2str(harm),'}',newline,'{\color{red}\bf\fontsize{12}\{X\}}',newline,'{\color{black}\bf\fontsize{12}Ho:',num2str(2*harm),newline,'{\color{blue}\bf\fontsize{12}MEX}','}'], 'texmode','on');
      | else
      |     disp(['{\color{black}\bf\fontsize{12}Hi:',num2str(harm),'}',newline,'{\color{red}\bf\fontsize{12}\{X\}}',newline,'{\color{black}\bf\fontsize{12}Ho:',num2str(harm),newline,'{\color{orange}\bf\fontsize{12}MEX}','}'], 'texmode','on');
      | end
      | 
      | %disp([newline,newline,newline,newline,newline,'{\color{black}\bf\fontsize{12}MEX}'],  'texmode','on');
      | 
      | 
      | 
      | %text(.95,.05,[newline,'{\bf\fontsize{12}H=',harm,'}'], 'horizontalAlignment', 'right', 'verticalAlignment','bottom','texmode','on')
  sMult_DQN2 : Subsystem  mask{HRM=1, HrmDbl=on, selHrm=on, selMat=zeros(3,6)}
      mask prompts: HRM "Harmonic order:"; HrmDbl "Double harmonics"; selHrm "Specific harmonics"; selMat "Select matrix [(1+HrmDbl)*N+1]:"
      mask init:
      | if(HrmDbl == 0 && selHrm == 0)
      |     HrmOpt = 0;
      | elseif(HrmDbl == 1 && selHrm == 0)
      |     HrmOpt = 1;
      | elseif(HrmDbl == 0 && selHrm == 1)
      |     HrmOpt = 2;
      | else
      |     HrmOpt = 3;
      | end
      | 
      | 
      | if(selHrm == 1)
      |    
      |     if(size(selMat,2) ~= 6)
      |        error('Invalid number of colums in the select matrix!'); 
      |     end
      |     if(size(selMat,1) ~= (1+HrmDbl)*HRM+1)
      |        error('Invalid number of rows in the select matrix!'); 
      |     end
      |     
      | end
      mask Callback selHrm:
      | EMT = get_param(gcb,'selHrm');
      | 
      | if(strcmp(EMT,'on'))
      |    set_param(gcb,'MaskVisibilities',{'on','on','on','on'});
      | else
      |    set_param(gcb,'MaskVisibilities',{'on','on','on','off'});
      | end
      mask Display:
      | %plot([0 1])
      | %port_label('input',1,'{X}');
      | %port_label('input',2,'{Y}');
      | %port_label('output',1,'{Z}');
      | 
      | port_label('input',1,'');
      | port_label('input',2,'');
      | port_label('output',1,'');
      | 
      | 
      | harm = str2num(get_param(gcb, 'HRM'));
      | HrmDbl = get_param(gcb, 'HrmDbl');
      | if(HrmDbl=="on")
      |     disp(['{\color{black}\bf\fontsize{12}Hi:',num2str(harm),'}',newline,'{\color{red}\bf\fontsize{12}\{X\}}',newline,'{\color{black}\bf\fontsize{12}Ho:',num2str(2*harm),newline,'{\color{blue}\bf\fontsize{12}MEX}',newline,'{\color{black}\bf\fontsize{12}MAT}','}'], 'texmode','on');
      | else
      |     disp(['{\color{black}\bf\fontsize{12}Hi:',num2str(harm),'}',newline,'{\color{red}\bf\fontsize{12}\{X\}}',newline,'{\color{black}\bf\fontsize{12}Ho:',num2str(harm),newline,'{\color{orange}\bf\fontsize{12}MEX}',newline,'{\color{black}\bf\fontsize{12}MAT}','}'], 'texmode','on');
      | end
      | 
      | %disp([newline,newline,newline,newline,newline,'{\color{black}\bf\fontsize{12}MEX}'],  'texmode','on');
      | 
      | 
      | 
      | %text(.95,.05,[newline,'{\bf\fontsize{12}H=',harm,'}'], 'horizontalAlignment', 'right', 'verticalAlignment','bottom','texmode','on')
  sMult_DQN_old : Subsystem  mask{HrmOrd=N, HrmDbl=on}
      mask prompts: HrmOrd "Harmonic order"; HrmDbl "Double harmonic?"
      mask Display:
      | %plot([0 1])
      | port_label('input',1,'{X}');
      | port_label('input',2,'{Y}');
      | port_label('output',1,'{Z}');
      | 
      | 
      | 
      | harm = str2num(get_param(gcb, 'HrmOrd'));
      | HrmDbl = get_param(gcb, 'HrmDbl');
      | if(HrmDbl=="on")
      |     disp(['{\color{black}\bf\fontsize{12}Hi:',num2str(harm),'}',newline,'{\color{red}\bf\fontsize{12}\{X\}}',newline,'{\color{black}\bf\fontsize{12}Ho:',num2str(2*harm),newline,'{\color{blue}\bf\fontsize{12}MEX}','}'], 'texmode','on');
      | else
      |     disp(['{\color{black}\bf\fontsize{12}Hi:',num2str(harm),'}',newline,'{\color{red}\bf\fontsize{12}\{X\}}',newline,'{\color{black}\bf\fontsize{12}Ho:',num2str(harm),newline,'{\color{orange}\bf\fontsize{12}MEX}','}'], 'texmode','on');
      | end
      | 
      | %disp([newline,newline,newline,newline,newline,'{\color{black}\bf\fontsize{12}MEX}'],  'texmode','on');
      | 
      | 
      | 
      | %text(.95,.05,[newline,'{\bf\fontsize{12}H=',harm,'}'], 'horizontalAlignment', 'right', 'verticalAlignment','bottom','texmode','on')
  sSumDQN : Subsystem  mask{HrmOrd=1}
      mask prompts: HrmOrd "Harmonic order:"
      mask Display:
      | %plot([0 1])
      | %port_label('input',1,'{X}');
      | %port_label('output',1,'{Z}');
      | 
      | port_label('input',1,'');
      | port_label('output',1,'');
      | 
      | harm = get_param(gcb, 'HrmOrd');
      | disp(['{\color{black}\bf\fontsize{12}Hi:',(harm),'}',newline,'{\color{red}\bf\fontsize{12}\{\Sigma\}}',newline,'{\color{black}\bf\fontsize{12}Ho:',(harm),'}',newline,'{\color{blue}\bf\fontsize{12}MEX}'], 'texmode','on');

== system DQN_Lib (conflicted copy 2023-11-25 154811)/Add_DQN ==
  X_DQN : Inport
  Y_DQN : Inport  Port=2
  Demux : Demux  Outputs=6
  Demux1 : Demux  Outputs=6
  MATLAB Function1 : MATLAB Function  TreatAsAtomicUnit=on  mask{N=HrmOrd, chkHrmLst=chkHrmLst, HrmLst=HrmLst}
      mask prompts: N "Harmonic order:"; chkHrmLst "Chosen harmonics"; HrmLst "Harmonic list:"
  Mux51 : Mux  Inputs=[(1)*HrmOrd+1,(1)*HrmOrd+1,(1)*HrmOrd+1,(1)*HrmOrd+1,(1)*HrmOrd+1,(1)*HrmOrd+1]
  Z_DQN : Outport
  wires:
  X_DQN/1 -> Demux/1
  Y_DQN/1 -> Demux1/1
  Mux51/1 -> Z_DQN/1
  MATLAB Function1/3(Zdz) -> Mux51/3
  MATLAB Function1/2(Zdn) -> Mux51/2
  MATLAB Function1/4(Zqp) -> Mux51/4
  MATLAB Function1/1(Zdp) -> Mux51/1
  MATLAB Function1/5(Zqn) -> Mux51/5
  MATLAB Function1/6(Zqz) -> Mux51/6
  Demux/1 -> MATLAB Function1/1(Xdp)
  Demux/2 -> MATLAB Function1/2(Xdn)
  Demux/3 -> MATLAB Function1/3(Xdz)
  Demux/4 -> MATLAB Function1/4(Xqp)
  Demux/5 -> MATLAB Function1/5(Xqn)
  Demux/6 -> MATLAB Function1/6(Xqz)
  Demux1/1 -> MATLAB Function1/7(Ydp)
  Demux1/2 -> MATLAB Function1/8(Ydn)
  Demux1/3 -> MATLAB Function1/9(Ydz)
  Demux1/4 -> MATLAB Function1/10(Yqp)
  Demux1/5 -> MATLAB Function1/11(Yqn)
  Demux1/6 -> MATLAB Function1/12(Yqz)

== system DQN_Lib (conflicted copy 2023-11-25 154811)/BACKUP ==
  Gain_DQNc_Mat1 : MATLAB Function  TreatAsAtomicUnit=on  mask{HRM=0, Rabc=zeros(3,3), chkInv=off}
      mask prompts: HRM "Harmonic order:"; Rabc "Line matrix [3x3]"; chkInv "Invert"
  Int_DQN_Mat : MATLAB Function  TreatAsAtomicUnit=on  mask{N=HrmOrd, dt=TimeStep, w=FreqRad, EMT=on, InitInt=Init}
      mask prompts: N "Order number:"; dt "Time step (s):"; w "Angular frequency (1/rad):"; InitInt "Initial conditions [1x6]:"
  Int_DQNc_Mat : MATLAB Function  TreatAsAtomicUnit=on  mask{N=1, dt=50e-6, w=2*pi*50, InitInt=zeros(3,1)}
      mask prompts: N "Order number:"; dt "Time step (s):"; w "Angular frequency (1/rad):"; InitInt "Initial conditions DC [3x1]:"
  Int_DQNc_Mat1 : MATLAB Function  TreatAsAtomicUnit=on  mask{N=1, dt=50e-6, w=2*pi*50, InitInt=[0; 0; 0], swFeed=off, R=1, iL=1}
      mask prompts: N "Order number:"; dt "Time step (s):"; w "Angular frequency (1/rad):"; InitInt "Initial conditions DC [3x1]:"; swFeed "Enable feedback"; R "Feedback parameter (Kr):"; iL "Feedback parameter (Ki):"
  MatMultDQN1 : MATLAB Function  Commented=on  TreatAsAtomicUnit=on  mask{H=1, R=[], chkInv=off}
      mask prompts: H "Harmonic order:"; R "Line matrix [3x3]"; chkInv "Invert?"

== system DQN_Lib (conflicted copy 2023-11-25 154811)/DQN2abc ==
  DQN : Inport
  th : Inport  Port=2
  DQn->ABC19 : MATLAB Function  TreatAsAtomicUnit=on  mask{N=HrmOrd}
      mask prompts: N "Harmonic order:"
  Demux46 : Demux  Outputs=6
  abc : Outport
  wires:
  DQn->ABC19/1(abc) -> abc/1
  DQN/1 -> Demux46/1
  th/1 -> DQn->ABC19/7(th)
  Demux46/1 -> DQn->ABC19/1(Xdp)
  Demux46/2 -> DQn->ABC19/2(Xdn)
  Demux46/3 -> DQn->ABC19/3(Xdz)
  Demux46/4 -> DQn->ABC19/4(Xqp)
  Demux46/5 -> DQn->ABC19/5(Xqn)
  Demux46/6 -> DQn->ABC19/6(Xqz)

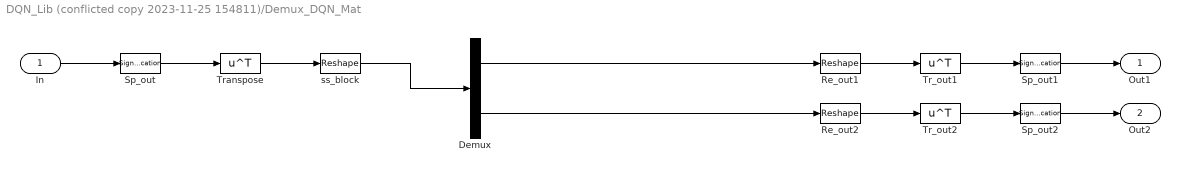
== system DQN_Lib (conflicted copy 2023-11-25 154811)/Demux_DQN_Mat ==
  In : Inport
  Demux : Demux  Outputs=[6,6]
  Re_out1 : Reshape  OutputDimensionality=Customize  OutputDimensions=[6,1]
  Re_out2 : Reshape  OutputDimensionality=Customize  OutputDimensions=[6,1]
  Sp_out : SignalSpecification  Dimensions=[2,6]
  Sp_out1 : SignalSpecification  Dimensions=[6,1]
  Sp_out2 : SignalSpecification  Dimensions=[6,1]
  Tr_out1 : Math  Operator=transpose
  Tr_out2 : Math  Operator=transpose
  Transpose : Math  Operator=transpose
  ss_block : Reshape  OutputDimensionality=Customize  OutputDimensions=[6,2*(1)]
  Out1 : Outport
  Out2 : Outport  Port=2
  wires:
  In/1 -> Sp_out/1
  Sp_out/1 -> Transpose/1
  Transpose/1 -> ss_block/1
  ss_block/1 -> Demux/1
  Demux/1 -> Re_out1/1
  Re_out1/1 -> Tr_out1/1
  Tr_out1/1 -> Sp_out1/1
  Sp_out1/1 -> Out1/1
  Demux/2 -> Re_out2/1
  Re_out2/1 -> Tr_out2/1
  Tr_out2/1 -> Sp_out2/1
  Sp_out2/1 -> Out2/1

== system DQN_Lib (conflicted copy 2023-11-25 154811)/Demux_DQNc_Mat ==
  In1 : Inport
  Sel1 : Selector  NumberOfDimensions=2  InputPortWidth=3  IndexOptions=Index vector (dialog),Select all  Indices=1:3, 1  OutputSizes=1
  Sel2 : Selector  NumberOfDimensions=2  InputPortWidth=3  IndexOptions=Index vector (dialog),Select all  Indices=4:6, 1  OutputSizes=1
  Out1 : Outport
  Out2 : Outport  Port=2
  wires:
  In1/1 -> Sel1/1, Sel2/1
  Sel1/1 -> Out1/1
  Sel2/1 -> Out2/1

== system DQN_Lib (conflicted copy 2023-11-25 154811)/Der_DQN ==
  X_DQN : Inport
  Demux : Demux  Outputs=6
  MATLAB Function3 : MATLAB Function  TreatAsAtomicUnit=on  mask{N=HrmOrd, w=FreqRad, Ts=Ts, EMT=EMT, SoftStart=sw_soft, chkHrmLst=chkHrmLst, HrmLst=HrmLst}
      mask prompts: N "Harmonic order:"; w "Frequency (rad/s):"; Ts "Time step (s):"; EMT "Enable EMT"; SoftStart "Soft start?"; chkHrmLst "Selected harmonics"; HrmLst "Harmonic list:"
  Mux51 : Mux  Inputs=[(1)*HrmOrd+1,(1)*HrmOrd+1,(1)*HrmOrd+1,(1)*HrmOrd+1,(1)*HrmOrd+1,(1)*HrmOrd+1]
  Z_DQN : Outport
  wires:
  X_DQN/1 -> Demux/1
  Mux51/1 -> Z_DQN/1
  Demux/3 -> MATLAB Function3/3(Xdz)
  Demux/2 -> MATLAB Function3/2(Xdn)
  Demux/4 -> MATLAB Function3/4(Xqp)
  Demux/1 -> MATLAB Function3/1(Xdp)
  Demux/5 -> MATLAB Function3/5(Xqn)
  Demux/6 -> MATLAB Function3/6(Xqz)
  MATLAB Function3/3(dZdz) -> Mux51/3
  MATLAB Function3/2(dZdn) -> Mux51/2
  MATLAB Function3/4(dZqp) -> Mux51/4
  MATLAB Function3/1(dZdp) -> Mux51/1
  MATLAB Function3/5(dZqn) -> Mux51/5
  MATLAB Function3/6(dZqz) -> Mux51/6
